simulink model "untitled"  (R2017a)
settings: Solver=ode45  StartTime=0.0  StopTime=0.0025  RelTol=1e-9
undefined symbols (not defined in the file): H, Tau1, Tau2, Tau3
libraries: dspmlti4 x12, simulink x1
settings Model: Creator=bhannigan  LastModifiedBy=bhannigan

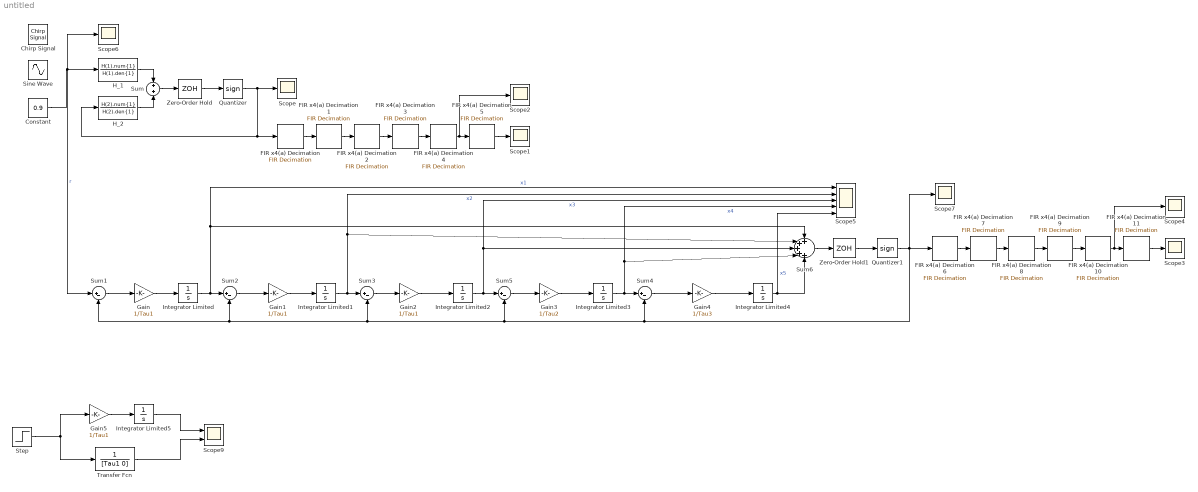
== system untitled ==
  Chirp Signal : simulink/Sources/Chirp Signal  f1=10  T=1  f2=15000
  Constant : Constant  Value=0.9
  FIR x4(a) Decimation{,1..9,11} (11 alike) : dspmlti4/FIR Decimation  FilterSource=Dialog parameters  h=fir1(31,0.15)  D=2  filtStruct=Direct form  FilterObject=Hm_firdecim  framing=Allow multirate processing  inputOffset=0  outputBufInitCond=0  roundingMode=Floor  overflowMode=off  firstCoeffDataTypeStr=Inherit: Same word length as input  firstCoeffMin=[]  firstCoeffMax=[]  firstCoeffLastDataTypeStr=Inherit: Same word length as input  accumDataTypeStr=Inherit: Same as product output  accumLastDataTypeStr=Inherit: Same as product output  outputMin=[]  outputMax=[]
  FIR x4(a) Decimation10 : dspmlti4/FIR Decimation  FilterSource=Dialog parameters  h=fir1(31,0.15)  D=4  filtStruct=Direct form  FilterObject=Hm_firdecim  framing=Allow multirate processing  inputOffset=0  outputBufInitCond=0  roundingMode=Floor  overflowMode=off  firstCoeffDataTypeStr=Inherit: Same word length as input  firstCoeffMin=[]  firstCoeffMax=[]  firstCoeffLastDataTypeStr=Inherit: Same word length as input  accumDataTypeStr=Inherit: Same as product output  accumLastDataTypeStr=Inherit: Same as product output  outputMin=[]  outputMax=[]
  Gain{,1..2,5} (4 alike) : Gain  Gain=1/Tau1
  Gain3 : Gain  Gain=1/Tau2
  Gain4 : Gain  Gain=1/Tau3
  H_1 : TransferFcn  Numerator=H(1).num{1}  Denominator=H(1).den{1}
  H_2 : TransferFcn  Numerator=H(2).num{1}  Denominator=H(2).den{1}
  Integrator Limited : Integrator  UpperSaturationLimit=3  LowerSaturationLimit=-3  WrappedStateUpperValue=3  WrappedStateLowerValue=-3
  Integrator Limited{1..4} (4 alike) : Integrator  LimitOutput=on  UpperSaturationLimit=3  LowerSaturationLimit=-3  WrappedStateUpperValue=3  WrappedStateLowerValue=-3
  Integrator Limited5 : Integrator  LimitOutput=on  UpperSaturationLimit=Inf  LowerSaturationLimit=-Inf
  Quantizer : Signum
  Quantizer1 : Signum
  Scope{,1..4,6..7} (7 alike) : Scope
  Scope5 : Scope  NumInputPorts=5
  Scope9 : Scope  NumInputPorts=2
  Sine Wave : Sin  Amplitude=0.5  Frequency=2*pi*20000  SampleTime=0
  Step : Step  Time=100e-12  SampleTime=0
  Sum : Sum  Inputs=+|+
  Sum{1..5} (5 alike) : Sum  Inputs=|+-
  Sum6 : Sum  Inputs=+++++
  Transfer Fcn : TransferFcn  Denominator=[Tau1 0]
  Zero-Order Hold : ZeroOrderHold  SampleTime=1/2.8224e6
  Zero-Order Hold1 : ZeroOrderHold  SampleTime=1/2.8224e6
  wires:
  H_2/1 -> Sum/2
  Constant/1 -> Scope6/1, Sum1/1, H_1/1  "r"
  Quantizer/1 -> Scope/1, FIR x4(a) Decimation/1, H_2/1
  Sum/1 -> Zero-Order Hold/1
  Zero-Order Hold/1 -> Quantizer/1
  FIR x4(a) Decimation5/1 -> Scope1/1
  FIR x4(a) Decimation/1 -> FIR x4(a) Decimation1/1
  FIR x4(a) Decimation1/1 -> FIR x4(a) Decimation2/1
  FIR x4(a) Decimation2/1 -> FIR x4(a) Decimation3/1
  FIR x4(a) Decimation3/1 -> FIR x4(a) Decimation4/1
  FIR x4(a) Decimation4/1 -> Scope2/1, FIR x4(a) Decimation5/1
  Sum1/1 -> Gain/1
  Sum2/1 -> Gain1/1
  Sum3/1 -> Gain2/1
  Integrator Limited2/1 -> Scope5/3, Sum6/3, Sum5/1  "x3"
  Sum5/1 -> Gain3/1
  Sum4/1 -> Gain4/1
  Integrator Limited3/1 -> Scope5/4, Sum6/4, Sum4/1  "x4"
  Integrator Limited1/1 -> Scope5/2, Sum6/2, Sum3/1  "x2"
  Integrator Limited/1 -> Sum6/1, Scope5/1, Sum2/1  "x1"
  Integrator Limited4/1 -> Scope5/5, Sum6/5  "x5"
  Sum6/1 -> Zero-Order Hold1/1
  Zero-Order Hold1/1 -> Quantizer1/1
  Quantizer1/1 -> Scope7/1, FIR x4(a) Decimation6/1, Sum2/2, Sum1/2, Sum3/2, Sum5/2, Sum4/2
  FIR x4(a) Decimation6/1 -> FIR x4(a) Decimation7/1
  FIR x4(a) Decimation9/1 -> FIR x4(a) Decimation10/1
  FIR x4(a) Decimation8/1 -> FIR x4(a) Decimation9/1
  FIR x4(a) Decimation7/1 -> FIR x4(a) Decimation8/1
  FIR x4(a) Decimation11/1 -> Scope3/1
  FIR x4(a) Decimation10/1 -> Scope4/1, FIR x4(a) Decimation11/1
  H_1/1 -> Sum/1
  Gain1/1 -> Integrator Limited1/1
  Gain/1 -> Integrator Limited/1
  Gain2/1 -> Integrator Limited2/1
  Gain3/1 -> Integrator Limited3/1
  Gain4/1 -> Integrator Limited4/1
  Step/1 -> Transfer Fcn/1, Gain5/1
  Gain5/1 -> Integrator Limited5/1
  Integrator Limited5/1 -> Scope9/1
  Transfer Fcn/1 -> Scope9/2
